simulink model "full_bridge_single_phase_inverter_sine_pwm"  (R2021a)
settings: Solver=ode4  StartTime=0.0  StopTime=0.1  FixedStep=1e-6  RelTol=1e-3
libraries: spsIGBTDiodeLib x4, spsCurrentMeasurementLib x1, spsDCVoltageSourceLib x1, spsSeriesRLCLoadLib x1, simulink x1, spsVoltageMeasurementLib x1, spspowerguiLib x1
settings Model: Creator=PRANAY KAMAL  LastModifiedBy=PRANAY KAMAL
settings DataIOCC: ReturnWorkspaceOutputs=off

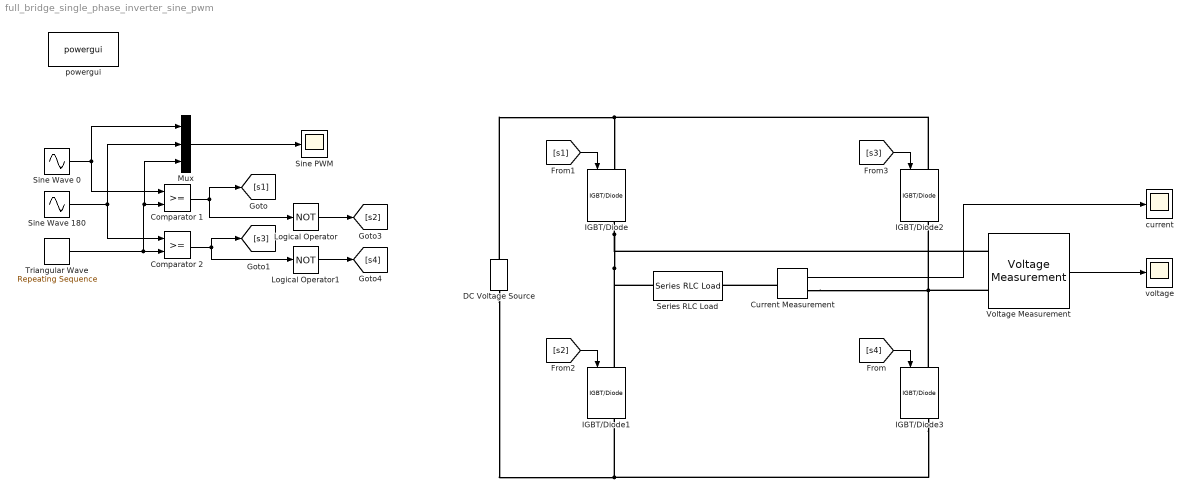
== system full_bridge_single_phase_inverter_sine_pwm ==
  Comparator 1 : RelationalOperator  OutDataTypeStr=boolean  RndMeth=Simplest
  Comparator 2 : RelationalOperator  OutDataTypeStr=boolean  RndMeth=Simplest
  Current Measurement : spsCurrentMeasurementLib/Current Measurement  PhasorSimulation=off  OutputType=Complex  PSBequivalent=0
  DC Voltage Source : spsDCVoltageSourceLib/DC Voltage Source  Amplitude=400  Measurements=None
  IGBT/Diode{,1..3} (4 alike) : spsIGBTDiodeLib/IGBT//Diode  Ron=1e-3  Rs=1e5  Cs=inf  Measurements=on
  Logical Operator : Logic  Operator=NOT  AllPortsSameDT=off  OutDataTypeStr=boolean
  Logical Operator1 : Logic  Operator=NOT  AllPortsSameDT=off  OutDataTypeStr=boolean
  Mux : Mux  Inputs=3
  Series RLC Load : spsSeriesRLCLoadLib/Series RLC Load  LConnTagsString=a  RConnTagsString=__new0  NominalVoltage=1000  NominalFrequency=50  ActivePower=10e3  InductivePower=500  CapacitivePower=0  Setx0=off  InitialVoltage=0  SetiL0=off  InitialCurrent=0  Measurements=Branch voltage and current  LoadType=constant Z
  Sine PWM : Scope
  Sine Wave 0 : Sin  Amplitude=0.8  Frequency=2*pi*60  SampleTime=0
  Sine Wave 180 : Sin  Amplitude=0.8  Frequency=2*pi*60  Phase=pi  SampleTime=0
  Triangular Wave : simulink/Sources/Repeating Sequence  rep_seq_t=[0 0.5 1]*[1/6000]  rep_seq_y=[1 -1 1]
  Voltage Measurement : spsVoltageMeasurementLib/Voltage Measurement  PhasorSimulation=off  OutputType=Complex  PSBequivalent=0
  current : Scope
  powergui : spspowerguiLib/powergui  Priority=1  SimulationMode=Continuous  SampleTime=50e-6  frequency=60  Iterations=50  frequencyindice=0  Pbase=100e6  ErrMax=1e-4  UnitsV=kV  UnitsW=MW  buscounter=0  FunctionMessages=off  echomessages=off  EnableUseOfTLC=off  CurrentSourceSwitches=off  DisableSnubberDevices=off  DisableRonSwitches=off  DisableVfSwitches=off  DisplayEquations=off  AutomaticDiscreteSolvers=off  SolverType=Tustin/Backward Euler (TBE)  Interpol=off  ExternalGateDelay=off  methode=off  Ts=100  x0status=blocks  SPID=on  SwTol=0  HookPort=off  NonlinearTolerance=1e-4  nMaxIteration=100  ContinueOnMaxIteration=off  RestoreLinks=warning  ResistiveCurrentMeasurement=off  Frange=[0:2:500]  Ylog=off  Xlog=on  ShowGrid=off  save=off  variable=ZData  structure=0  ZoomFFT=off  StartTime=0.0  cycles=1  DisplayStyle=1  fundamental=60  FreqAxis=off  MaxFrequency=1000  frequencyindicesteady=1  RmsSteady=1  display=off
  voltage : Scope
  wires:
  [s3] -> IGBT/Diode2/1
  [s4] -> IGBT/Diode3/1
  Voltage Measurement/1 -> voltage/1
  [s2] -> IGBT/Diode1/1
  Current Measurement/1 -> current/1
  [s1] -> IGBT/Diode/1
  Comparator 2/1 -> Logical Operator1/1, [s3]
  Mux/1 -> Sine PWM/1
  Triangular Wave/1 -> Comparator 2/2, Mux/3, Comparator 1/2
  Sine Wave 0/1 -> Mux/1, Comparator 1/1
  Comparator 1/1 -> Logical Operator/1, [s1]
  Sine Wave 180/1 -> Mux/2, Comparator 2/1
  Logical Operator/1 -> [s2]
  Logical Operator1/1 -> [s4]
  connections:
  DC Voltage Source/RConn1 -- IGBT/Diode2/LConn1 -- IGBT/Diode/LConn1
  IGBT/Diode/RConn1 -- IGBT/Diode1/LConn1 -- Series RLC Load/LConn1 -- Voltage Measurement/LConn1
  IGBT/Diode3/LConn1 -- IGBT/Diode2/RConn1 -- Voltage Measurement/LConn2 -- Current Measurement/RConn1
  DC Voltage Source/LConn1 -- IGBT/Diode1/RConn1 -- IGBT/Diode3/RConn1
  Current Measurement/LConn1 -- Series RLC Load/RConn1
